simulink model "optimizeSim"  (R2020b)
settings: Solver=VariableStepAuto  StartTime=0.0  StopTime=inf  RelTol=1e-3
libraries: simulink x1
settings Model: Creator=e406594  LastModifiedBy=e406594

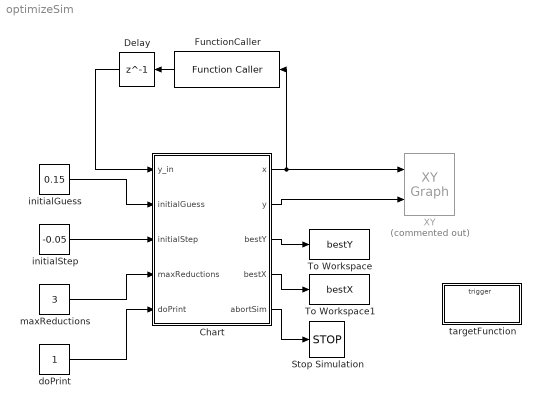
== system optimizeSim ==
  Chart : Stateflow chart  TreatAsAtomicUnit=on
  Delay : Delay  DelayLength=1
  FunctionCaller : FunctionCaller  FunctionPrototype=y = f(x)  InputArgumentSpecifications=<Enter example>  OutputArgumentSpecifications=<Enter example>
  Stop Simulation : Stop
  To Workspace : ToWorkspace  VariableName=bestY  SampleTime=-1
      settings: MaxDataPoints=1  Save2DSignal=2-D array (concatenate along first dimension)
  To Workspace1 : ToWorkspace  VariableName=bestX  SampleTime=-1
      settings: MaxDataPoints=1  Save2DSignal=2-D array (concatenate along first dimension)
  XY : simulink/Sinks/XY Graph  Commented=on  xmin=-1  xmax=4  ymin=-3  ymax=5  st=-1
  doPrint : Constant
  initialGuess : Constant  Value=0.15
  initialStep : Constant  Value=-0.05
  maxReductions : Constant  Value=3
  targetFunction : Subsystem  TreatAsAtomicUnit=on
  wires:
  Chart/4(bestX) -> To Workspace1/1
  doPrint/1 -> Chart/5(doPrint)
  maxReductions/1 -> Chart/4(maxReductions)
  Chart/1(x) -> XY/1, FunctionCaller/1
  initialGuess/1 -> Chart/2(initialGuess)
  Chart/3(bestY) -> To Workspace/1
  initialStep/1 -> Chart/3(initialStep)
  Chart/5(abortSim) -> Stop Simulation/1
  FunctionCaller/1 -> Delay/1
  Delay/1 -> Chart/1(y_in)
  Chart/2(y) -> XY/2

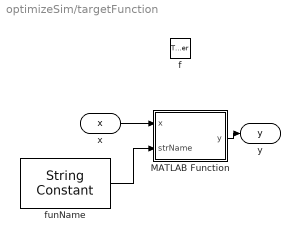
== system optimizeSim/targetFunction ==
  f : TriggerPort  TriggerType=function-call  IsSimulinkFunction=on  FunctionName=f  FunctionVisibility=scoped  VariantControl=(inherit)
  MATLAB Function : MATLAB Function  TreatAsAtomicUnit=on
  funName : StringConstant  String="\"optS1NozzExit\""
  x : ArgIn  DisableCoverage=on  ArgumentName=x
  y : ArgOut  DisableCoverage=on  ArgumentName=y
  wires:
  x/1 -> MATLAB Function/1(x)
  MATLAB Function/1(y) -> y/1
  funName/1 -> MATLAB Function/2(strName)

== matlab function optimizeSim/targetFunction/MATLAB Function ==
  data: x input; y output; strName input
function y = fcn(x,strName)
persistent setup
y = 0;
% y = -x^2;


y = feval(strName,x);
end

== stateflow chart optimizeSim/Chart ==
  state Start
    entry:
    x = initialGuess;
  state Exit
    entry:
    if doPrint
    fprintf('\nBest:\n');
    fprintf('x: %+f\ty: %+f\n',bestX,bestY);
    end
    y = 0;
    abortSim = true;
  state Setup
    entry:
    y = y_in;
    bestX = x;
    bestY = y;
    step = initialStep;
    changeDirection = 1;
    reductions = 0;
    abortSim = false;
    if doPrint
    fprintf('x: %+f\ty: %+f\n',x,y);
    end
  state StepX
    x = x + step;
  state CalcNew
    entry:
    y = y_in;
    if doPrint
    fprintf('x: %+f\ty: %+f\n',x,y);
    end
  state NewBest
    entry:
    bestX = x;
    bestY = y;
    changeDirection = 0;
  state ChangeDir
    entry:
    step = -step;
    x = x + step;
    changeDirection = changeDirection + 1;
  state Reduction
    entry:
    reductions = reductions + 1;
    changeDirection = 1;
    step = step / stepReduction;
  state Overshot
    entry:
    overshoot = x;
    x = x - step;
    y = bestY;
    changeDirection = 1;
    step = step / stepReduction;
    reductions = reductions + 1;
  (default) -> Start
  Start -> Setup
  (junction 50) -> Exit [order 1] : [reductions > maxReductions]{x = bestX;}
  Setup -> StepX
  (junction 50) -> StepX [order 2]
  (junction 58) -> (junction 50)
  (junction 53) -> (junction 58)
  NewBest -> StepX
  ChangeDir -> (junction 50) [order 2]
  Reduction -> (junction 58)
  (junction 55) -> (junction 53)
  StepX -> CalcNew
  CalcNew -> NewBest [order 1] : [y > bestY]
  CalcNew -> ChangeDir [order 2] : [changeDirection > 0]
  ChangeDir -> Reduction [order 1] : [changeDirection > 2]
  CalcNew -> Overshot [order 3]
  Overshot -> (junction 55)
  data: y_in input; x output; y output; step local; bestY output; bestX output; overshoot local; stepReduction local =5; changeDirection local; reductions local; initialGuess input; initialStep input; maxReductions input; doPrint input; abortSim output
